simulink model "AntriebeW_V2mdl"  (Simulink 7.6)
settings: Solver=ode45  StartTime=0.0  StopTime=SimulTime  RelTol=1e-3
values from neighbouring files (symbols this model uses):
  hsp = 200    [ParamtersAntriebeW.m]
  Kraft = 5    [ParamtersAntriebeW.m]
  m = 30    [ParamtersAntriebeW.m]
  r = 0.2    [ParamtersAntriebeW.m]
  Vorschub = 5    [ParamtersAntriebeW.m]
undefined symbols (not defined in the file or in its folder): MainDrive
settings Model: Creator=Coni  LastModifiedBy=conid

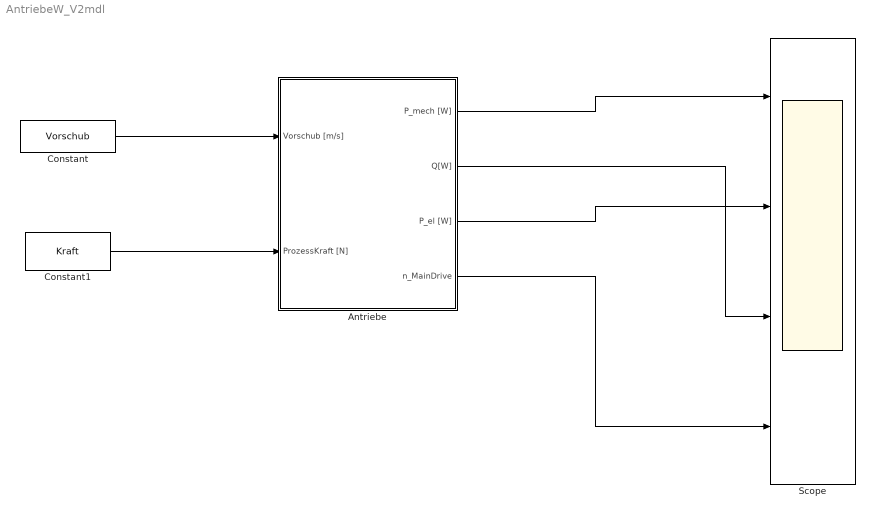
== system AntriebeW_V2mdl ==
  Antriebe : Subsystem  TreatAsAtomicUnit=on
  Constant : Constant  Value=Vorschub
  Constant1 : Constant  Value=Kraft
  Scope : Scope  NumInputPorts=4
      settings: TimeRange=4  YMin=39520~2.3624e+012~2.3624e+012~1.7595e-008  YMax=43680~2.3643e+012~2.3643e+012~1.7609e-008
  wires:
  Constant/1 -> Antriebe/1(Vorschub [m/s])
  Constant1/1 -> Antriebe/2(ProzessKraft [N])
  Antriebe/1(P_mech [W]) -> Scope/1
  Antriebe/3(P_el [W]) -> Scope/2
  Antriebe/2(Q[W]) -> Scope/3
  Antriebe/4(n_MainDrive) -> Scope/4

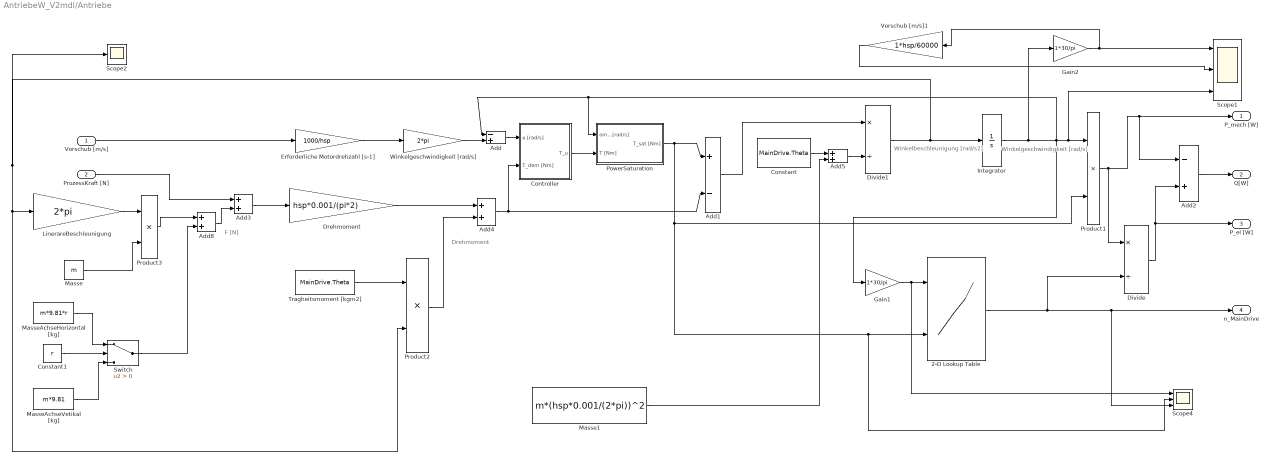
== system AntriebeW_V2mdl/Antriebe ==
  note: Winkelgeschwindigkeit [rad/s]
  note: Drehmoment
  note: F [N]
  note: Winkelbeschleunigung [rad/s2]
  Vorschub [m/s] : Inport
  ProzessKraft [N] : Inport  Port=2
  2-D Lookup Table : Lookup_n-D  BreakpointsForDimension1=MainDrive.Tabelomega  BreakpointsForDimension2=MainDrive.TabelM  BreakpointsForDimension1Min=[0]  BreakpointsForDimension2Min=[0]  BreakpointsForDimension1Max=[3000]  BreakpointsForDimension2Max=[9.5]  Table=MainDrive.Tabeleta  TableMin=[0]  TableMax=[1]  InterpMethod=Cubic spline  ExtrapMethod=Cubic spline  OutMin=[0]  OutMax=[1]  RndMeth=Simplest  InputSameDT=on
  Add : Sum  Inputs=-+
  Add1 : Sum  Inputs=+-
  Add2 : Sum  Inputs=-+
  Add{3..5,8} (4 alike) : Sum
  Constant : Constant  Value=MainDrive.Theta
  Constant1 : Constant  Value=r
  Controller : Subsystem  TreatAsAtomicUnit=on
  Divide : Product  Inputs=*/
  Divide1 : Product  Inputs=*/
  Drehmoment : Gain  Gain=hsp*0.001/(pi*2)
  Erforderliche Motordrehzahl [s-1] : Gain  Gain=1000/hsp
  Gain1 : Gain  Gain=1*30/pi
  Gain2 : Gain  Gain=1*30/pi
  Integrator : Integrator
  LinerareBeschleunigung : Gain  Gain=2*pi
  Masse : Constant  Value=m
  Masse1 : Constant  Value=m*(hsp*0.001/(2*pi))^2
  MasseAchseHorizontal [kg] : Constant  Value=m*9.81*r
  MasseAchseVetikal [kg] : Constant  Value=m*9.81
  PowerSaturation : Subsystem  TreatAsAtomicUnit=on
  Product1 : Product  RndMeth=Zero
  Product2 : Product  RndMeth=Zero
  Product3 : Product  RndMeth=Zero
  Scope1 : Scope  NumInputPorts=3
      settings: TimeRange=4  YMin=-5~-5~-5  YMax=5~5~5  SaveName=ScopeData2
  Scope2 : Scope
      settings: TimeRange=20  YMin=-2  YMax=6
  Scope4 : Scope  NumInputPorts=3
      settings: TimeRange=200  YMin=-1~-5~-5  YMax=1.5~5~5  SaveName=ScopeData3
  Switch : Switch  Criteria=u2 > Threshold
  Tragheitsmoment [kgm2] : Constant  Value=MainDrive.Theta
  Vorschub [m/s]1 : Gain  Gain=1*hsp/60000
  Winkelgeschwindigkeit [rad/s] : Gain  Gain=2*pi
  P_mech [W] : Outport
  Q[W] : Outport  Port=2
  P_el [W] : Outport  Port=3
  n_MainDrive : Outport  Port=4
  wires:
  Add/1 -> Controller/1(e [rad/s])
  Controller/1(T_u) -> PowerSaturation/2(T [Nm])
  PowerSaturation/1(T_sat [Nm]) -> Add1/1, Product1/2, 2-D Lookup Table/2, Scope4/2
  Divide1/1 -> Integrator/1, Product2/2, LinerareBeschleunigung/1, Scope2/1
  Integrator/1 -> Product1/1, Scope1/3, Add/1, PowerSaturation/1(omega [rad/s]), Gain1/1, Gain2/1
  Product1/1 -> Divide/1, P_mech [W]/1, Add2/1
  Add2/1 -> Q[W]/1
  Divide/1 -> Add2/2, P_el [W]/1
  2-D Lookup Table/1 -> Divide/2, n_MainDrive/1, Scope4/3
  Gain1/1 -> 2-D Lookup Table/1, Scope4/1
  Erforderliche Motordrehzahl [s-1]/1 -> Winkelgeschwindigkeit [rad/s]/1
  Winkelgeschwindigkeit [rad/s]/1 -> Add/2
  Add1/1 -> Divide1/1
  Add3/1 -> Drehmoment/1
  Add4/1 -> Add1/2, Controller/2(T_dem [Nm])
  Drehmoment/1 -> Add4/1
  ProzessKraft [N]/1 -> Add3/1
  Add5/1 -> Divide1/2
  Constant/1 -> Add5/1
  Tragheitsmoment [kgm2]/1 -> Product2/1
  Product2/1 -> Add4/2
  Gain2/1 -> Scope1/1, Vorschub [m/s]1/1
  MasseAchseHorizontal [kg]/1 -> Switch/1
  MasseAchseVetikal [kg]/1 -> Switch/3
  Constant1/1 -> Switch/2
  Vorschub [m/s]/1 -> Erforderliche Motordrehzahl [s-1]/1
  Vorschub [m/s]1/1 -> Scope1/2
  Masse1/1 -> Add5/2
  Add8/1 -> Add3/2
  Switch/1 -> Add8/2
  Masse/1 -> Product3/2
  Product3/1 -> Add8/1
  LinerareBeschleunigung/1 -> Product3/1

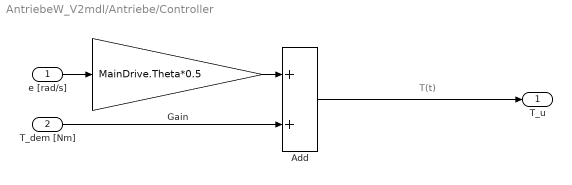
== system AntriebeW_V2mdl/Antriebe/Controller ==
  note: T(t)
  e [rad/s] : Inport
  T_dem [Nm] : Inport  Port=2
  Add : Sum
  Gain : Gain  Gain=MainDrive.Theta*0.5
  T_u : Outport
  wires:
  Add/1 -> T_u/1
  T_dem [Nm]/1 -> Add/2
  Gain/1 -> Add/1
  e [rad/s]/1 -> Gain/1

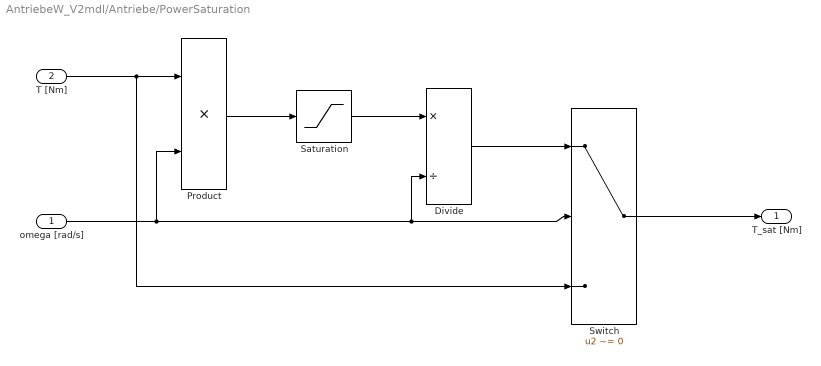
== system AntriebeW_V2mdl/Antriebe/PowerSaturation ==
  omega [rad/s] : Inport
  T [Nm] : Inport  Port=2
  Divide : Product  Inputs=*/
  Product : Product  RndMeth=Zero
  Saturation : Saturate  UpperLimit=MainDrive.Pmax  LowerLimit=-MainDrive.Pmax  ZeroCross=off
  Switch : Switch  Criteria=u2 ~= 0
  T_sat [Nm] : Outport
  wires:
  Product/1 -> Saturation/1
  Saturation/1 -> Divide/1
  Divide/1 -> Switch/1
  Switch/1 -> T_sat [Nm]/1
  T [Nm]/1 -> Product/1, Switch/3
  omega [rad/s]/1 -> Switch/2, Divide/2, Product/2
